simulink model "systemtotal"  (Simulink 8.5)
settings: Solver=ode23tb  SolverMode=SingleTasking  StartTime=0.0  StopTime=0.15  RelTol=1e-3  AbsTol=20e-6
undefined symbols (not defined in the file or in its folder): aux, den, dx, num, Time
libraries: powerlib x43, elements x5
(part 2 of 2)

== system systemtotal/Signal Processinng/DAB+OC I/OC1 ==
  note: v(t) is a vector
      | with width N1
  note: v_ort is
      | a complex number
  x : Inport
  OC filter : S-Function  FunctionName=oc1  Parameters=tfilt, rfilt, ifilt, tlen, N1
  dq : Outport  InitialOutput=0
  wires:
  x/1 -> OC filter/1
  OC filter/1 -> dq/1

== system systemtotal/Signal Processinng/DAB+OC I/OC2 ==
  note: v(t) is a vector
      | with width N1
  note: v_ort is
      | a complex number
  x : Inport
  OC filter : S-Function  FunctionName=oc1  Parameters=tfilt, rfilt, ifilt, tlen, N1
  dq : Outport  InitialOutput=0
  wires:
  x/1 -> OC filter/1
  OC filter/1 -> dq/1

== system systemtotal/Signal Processinng/DAB+OC I/OC3 ==
  note: v(t) is a vector
      | with width N1
  note: v_ort is
      | a complex number
  x : Inport
  OC filter : S-Function  FunctionName=oc1  Parameters=tfilt, rfilt, ifilt, tlen, N1
  dq : Outport  InitialOutput=0
  wires:
  x/1 -> OC filter/1
  OC filter/1 -> dq/1

== system systemtotal/Signal Processinng/DAB+OC V/DAB ==
  a : Inport
  A-D & Buffer : S-Function  FunctionName=dab2  Parameters=winsize,fs,dx,resdis
  Analog Filter : TransferFcn  Numerator=num  Denominator=den
  Gain : Gain  Gain=G  SaturateOnIntegerOverflow=on  OutDataTypeStr=Inherit: Same as input  ParamDataTypeStr=Inherit: Same as input
  Zero-Order Hold : ZeroOrderHold  SampleTime=1/fs
  d : Outport  InitialOutput=[zeros(winsize,1)]
  wires:
  A-D & Buffer/1 -> d/1
  a/1 -> Analog Filter/1
  Zero-Order Hold/1 -> A-D & Buffer/1
  Gain/1 -> Zero-Order Hold/1
  Analog Filter/1 -> Gain/1

== system systemtotal/Signal Processinng/DAB+OC V/DAB1 ==
  a : Inport
  A-D & Buffer : S-Function  FunctionName=dab2  Parameters=winsize,fs,dx,resdis
  Analog Filter : TransferFcn  Numerator=num  Denominator=den
  Gain : Gain  Gain=G  SaturateOnIntegerOverflow=on  OutDataTypeStr=Inherit: Same as input  ParamDataTypeStr=Inherit: Same as input
  Zero-Order Hold : ZeroOrderHold  SampleTime=1/fs
  d : Outport  InitialOutput=[zeros(winsize,1)]
  wires:
  A-D & Buffer/1 -> d/1
  a/1 -> Analog Filter/1
  Zero-Order Hold/1 -> A-D & Buffer/1
  Gain/1 -> Zero-Order Hold/1
  Analog Filter/1 -> Gain/1

== system systemtotal/Signal Processinng/DAB+OC V/DAB2 ==
  a : Inport
  A-D & Buffer : S-Function  FunctionName=dab2  Parameters=winsize,fs,dx,resdis
  Analog Filter : TransferFcn  Numerator=num  Denominator=den
  Gain : Gain  Gain=G  SaturateOnIntegerOverflow=on  OutDataTypeStr=Inherit: Same as input  ParamDataTypeStr=Inherit: Same as input
  Zero-Order Hold : ZeroOrderHold  SampleTime=1/fs
  d : Outport  InitialOutput=[zeros(winsize,1)]
  wires:
  A-D & Buffer/1 -> d/1
  a/1 -> Analog Filter/1
  Zero-Order Hold/1 -> A-D & Buffer/1
  Gain/1 -> Zero-Order Hold/1
  Analog Filter/1 -> Gain/1

== system systemtotal/Signal Processinng/DAB+OC V/OC ==
  note: v(t) is a vector
      | with width N1
  note: v_ort is
      | a complex number
  x : Inport
  OC filter : S-Function  FunctionName=oc1  Parameters=tfilt, rfilt, ifilt, tlen, N1
  dq : Outport  InitialOutput=0
  wires:
  x/1 -> OC filter/1
  OC filter/1 -> dq/1

== system systemtotal/Signal Processinng/DAB+OC V/OC1 ==
  note: v(t) is a vector
      | with width N1
  note: v_ort is
      | a complex number
  x : Inport
  OC filter : S-Function  FunctionName=oc1  Parameters=tfilt, rfilt, ifilt, tlen, N1
  dq : Outport  InitialOutput=0
  wires:
  x/1 -> OC filter/1
  OC filter/1 -> dq/1

== system systemtotal/Signal Processinng/DAB+OC V/OC2 ==
  note: v(t) is a vector
      | with width N1
  note: v_ort is
      | a complex number
  x : Inport
  OC filter : S-Function  FunctionName=oc1  Parameters=tfilt, rfilt, ifilt, tlen, N1
  dq : Outport  InitialOutput=0
  wires:
  x/1 -> OC filter/1
  OC filter/1 -> dq/1

== system systemtotal/Signal Processinng/DAB+OC V/OC3 ==
  note: v(t) is a vector
      | with width N1
  note: v_ort is
      | a complex number
  x : Inport
  OC filter : S-Function  FunctionName=oc1  Parameters=tfilt, rfilt, ifilt, tlen, N1
  dq : Outport  InitialOutput=0
  wires:
  x/1 -> OC filter/1
  OC filter/1 -> dq/1

== system systemtotal/Signal Processinng/DAB+OC V/OC4 ==
  note: v(t) is a vector
      | with width N1
  note: v_ort is
      | a complex number
  x : Inport
  OC filter : S-Function  FunctionName=oc1  Parameters=tfilt, rfilt, ifilt, tlen, N1
  dq : Outport  InitialOutput=0
  wires:
  x/1 -> OC filter/1
  OC filter/1 -> dq/1

== system systemtotal/Signal Processinng/DAB+OC V/OC5 ==
  note: v(t) is a vector
      | with width N1
  note: v_ort is
      | a complex number
  x : Inport
  OC filter : S-Function  FunctionName=oc1  Parameters=tfilt, rfilt, ifilt, tlen, N1
  dq : Outport  InitialOutput=0
  wires:
  x/1 -> OC filter/1
  OC filter/1 -> dq/1
